simulink model "NoDifferentialControl"  (R2024b)
settings: configuration reference "VehicleFixed10ms" (kept outside this file)
settings Model: DataDictionary=VirtualVehicleTemplate.sldd  ModifiedByFormat=The MathWorks, Inc.  Creator=The MathWorks, Inc.  LastModifiedBy=The MathWorks, Inc.
settings ConfigSetRef: SourceName=VehicleFixed10ms

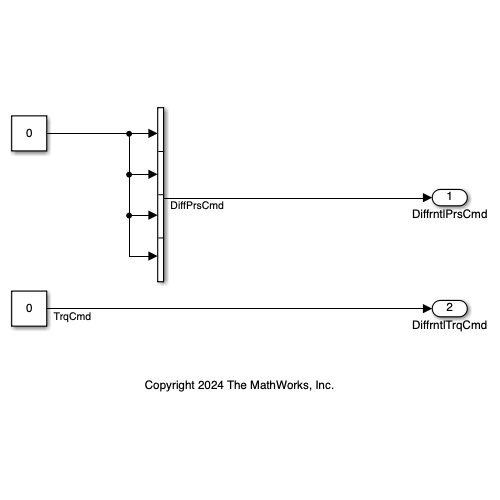
[thumbnail: Simulink's stored preview of the top-level diagram]
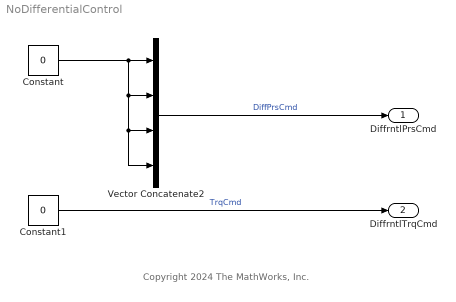
== system NoDifferentialControl ==
  note: Copyright 2024 The MathWorks, Inc.
  Constant : Constant  Value=0  SampleTime=-1
  Constant1 : Constant  Value=0  SampleTime=-1
  Vector Concatenate2 : Concatenate  NumInputs=4
  DiffrntlPrsCmd : Outport  VectorParamsAs1DForOutWhenUnconnected=off
  DiffrntlTrqCmd : Outport  Port=2  VectorParamsAs1DForOutWhenUnconnected=off
  wires:
  Vector Concatenate2/1 -> DiffrntlPrsCmd/1  "DiffPrsCmd"
  Constant1/1 -> DiffrntlTrqCmd/1  "TrqCmd"
  Constant/1 -> Vector Concatenate2/2, Vector Concatenate2/3, Vector Concatenate2/4, Vector Concatenate2/1
